simulink model "my_model"  (R2024a)
settings: Solver=VariableStepAuto  StartTime=0.0  StopTime=10.0  RelTol=1e-3
undefined symbols (not defined in the file): Kd, Kp, st0
settings Model: Creator=Qi Zhang  LastModifiedBy=dixiao
settings ConfigComp: CovBoundaryAbsTol=1.0e-5

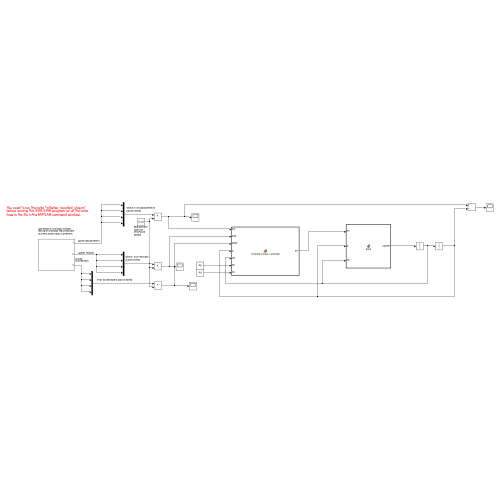
[thumbnail: Simulink's stored preview of the top-level diagram]
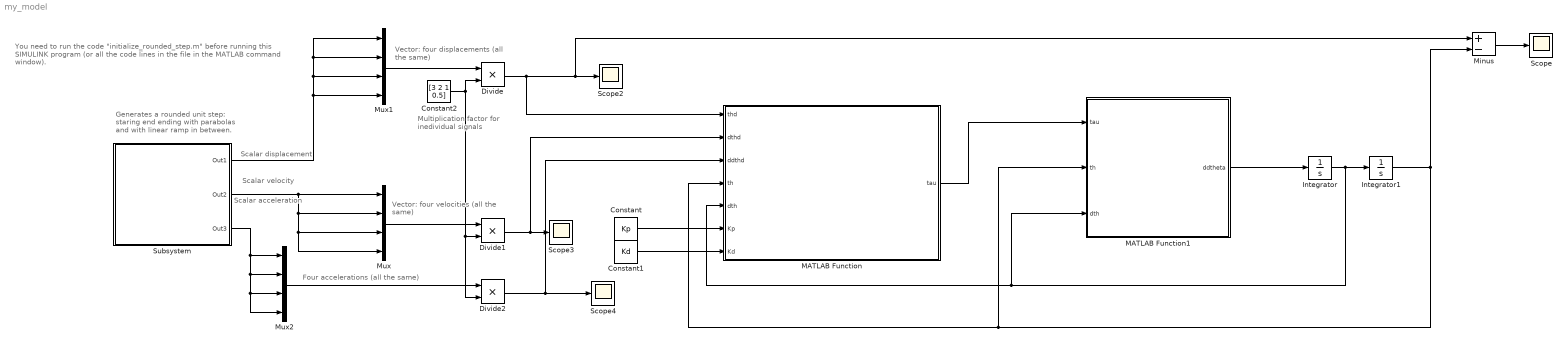
== system my_model ==
  note: You need to run the code "initialize_rounded_step.m"
      | before running this SIMULINK program (or all the code
      | lines in the file in the MATLAB command window).
  note: Generates a rounded unit step:
      | staring end ending with parabolas
      | and with linear ramp in between.
  note: Scalar velocity
  note: Four accelerations (all the same)
  note: Vector: four displacements
      | (all the same)
  note: Vector: four velocities
      | (all the same)
  note: Scalar displacement
  note: Multiplication
      | factor for
      | inedividual
      | signals
  note: Scalar
      | acceleration
  Constant : Constant  Value=Kp
  Constant1 : Constant  Value=Kd
  Constant2 : Constant  Value=[3 2 1 0.5]
  Divide : Product  Inputs=**
  Divide1 : Product  Inputs=**
  Divide2 : Product  Inputs=**
  Integrator : Integrator  InitialCondition=[0;0;0;0]
  Integrator1 : Integrator  InitialCondition=[0;0;0;0]
  MATLAB Function : MATLAB Function  TreatAsAtomicUnit=on
  MATLAB Function1 : MATLAB Function  TreatAsAtomicUnit=on
  Minus : Sum  Inputs=+-
  Mux : Mux
  Mux1 : Mux
  Mux2 : Mux
  Scope{,2..4} (4 alike) : Scope
  Subsystem : Subsystem
  wires:
  Subsystem/3(Out3) -> Mux2/2, Mux2/3, Mux2/4, Mux2/1
  Constant2/1 -> Divide2/2, Divide1/2, Divide/2
  Subsystem/2(Out2) -> Mux/4, Mux/3, Mux/2, Mux/1
  Mux1/1 -> Divide/1
  Divide/1 -> MATLAB Function/1(thd), Minus/1, Scope2/1
  Divide2/1 -> MATLAB Function/3(ddthd), Scope4/1
  Mux2/1 -> Divide2/1
  Mux/1 -> Divide1/1
  Subsystem/1(Out1) -> Mux1/1, Mux1/2, Mux1/3, Mux1/4
  Divide1/1 -> MATLAB Function/2(dthd), Scope3/1
  MATLAB Function1/1(ddtheta) -> Integrator/1
  Integrator/1 -> MATLAB Function1/3(dth), MATLAB Function/5(dth), Integrator1/1
  Constant/1 -> MATLAB Function/6(Kp)
  Constant1/1 -> MATLAB Function/7(Kd)
  Integrator1/1 -> Minus/2, MATLAB Function1/2(th), MATLAB Function/4(th)
  MATLAB Function/1(tau) -> MATLAB Function1/1(tau)
  Minus/1 -> Scope/1

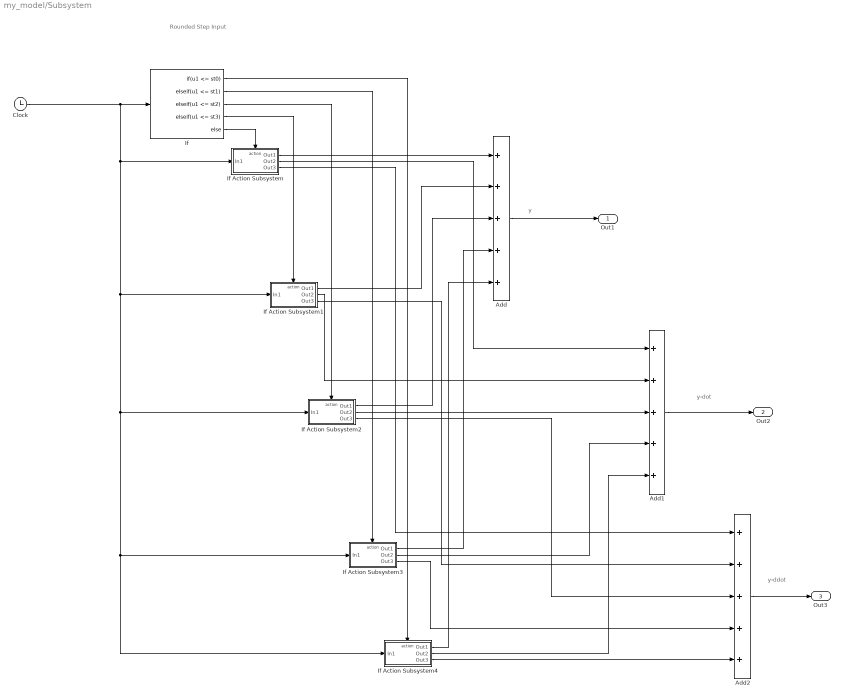
== system my_model/Subsystem ==
  note: Rounded Step Input
  note: y-ddot
  note: y-dot
  note: y
  Add : Sum  Inputs=+++++
  Add1 : Sum  Inputs=+++++
  Add2 : Sum  Inputs=+++++
  Clock : Clock
  If : If  IfExpression=u1 <= st0  ElseIfExpressions=u1 <= st1, u1 <= st2, u1 <= st3
  If Action Subsystem : Subsystem  TreatAsAtomicUnit=on
  If Action Subsystem1 : Subsystem  TreatAsAtomicUnit=on
  If Action Subsystem2 : Subsystem  TreatAsAtomicUnit=on
  If Action Subsystem3 : Subsystem  TreatAsAtomicUnit=on
  If Action Subsystem4 : Subsystem  TreatAsAtomicUnit=on
  Out1 : Outport
  Out2 : Outport  Port=2
  Out3 : Outport  Port=3
  wires:
  If Action Subsystem1/1(Out1) -> Add/2
  If/5 -> If Action Subsystem/Action
  If/3 -> If Action Subsystem2/Action
  If/2 -> If Action Subsystem3/Action
  If Action Subsystem/1(Out1) -> Add/1
  If Action Subsystem4/1(Out1) -> Add/5
  If/4 -> If Action Subsystem1/Action
  If/1 -> If Action Subsystem4/Action
  If Action Subsystem3/1(Out1) -> Add/4
  If Action Subsystem2/1(Out1) -> Add/3
  Add/1 -> Out1/1
  Add1/1 -> Out2/1
  Add2/1 -> Out3/1
  Clock/1 -> If Action Subsystem4/1(In1), If Action Subsystem3/1(In1), If Action Subsystem2/1(In1), If Action Subsystem1/1(In1), If Action Subsystem/1(In1), If/1
  If Action Subsystem/2(Out2) -> Add1/1
  If Action Subsystem/3(Out3) -> Add2/1
  If Action Subsystem1/2(Out2) -> Add1/2
  If Action Subsystem1/3(Out3) -> Add2/2
  If Action Subsystem2/2(Out2) -> Add1/3
  If Action Subsystem2/3(Out3) -> Add2/3
  If Action Subsystem3/3(Out3) -> Add2/4
  If Action Subsystem3/2(Out2) -> Add1/4
  If Action Subsystem4/2(Out2) -> Add1/5
  If Action Subsystem4/3(Out3) -> Add2/5

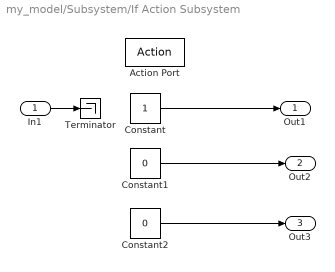
== system my_model/Subsystem/If Action Subsystem ==
  In1 : Inport
  Action Port : ActionPort  ActionPortLabel=else
  Constant : Constant
  Constant1 : Constant  Value=0
  Constant2 : Constant  Value=0
  Terminator : Terminator
  Out1 : Outport  OutputWhenDisabled=reset  InitialOutput=0
  Out2 : Outport  Port=2  OutputWhenDisabled=reset  InitialOutput=0
  Out3 : Outport  Port=3
  wires:
  Constant/1 -> Out1/1
  In1/1 -> Terminator/1
  Constant1/1 -> Out2/1
  Constant2/1 -> Out3/1

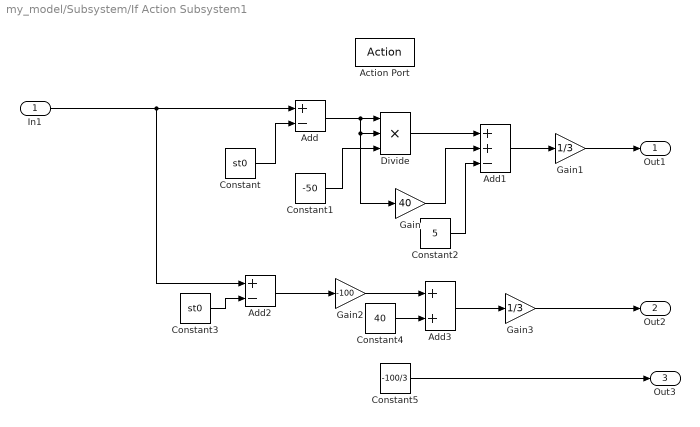
== system my_model/Subsystem/If Action Subsystem1 ==
  In1 : Inport
  Action Port : ActionPort  ActionPortLabel=elseif( u1 <= st3)
  Add : Sum  Inputs=+-
  Add1 : Sum  Inputs=++-
  Add2 : Sum  Inputs=+-
  Add3 : Sum
  Constant : Constant  Value=st0
  Constant1 : Constant  Value=-50
  Constant2 : Constant  Value=5
  Constant3 : Constant  Value=st0
  Constant4 : Constant  Value=40
  Constant5 : Constant  Value=-100/3
  Divide : Product  Inputs=***
  Gain : Gain  Gain=40
  Gain1 : Gain  Gain=1/3
  Gain2 : Gain  Gain=-100
  Gain3 : Gain  Gain=1/3
  Out1 : Outport  OutputWhenDisabled=reset  InitialOutput=0
  Out2 : Outport  Port=2  OutputWhenDisabled=reset  InitialOutput=0
  Out3 : Outport  Port=3  OutputWhenDisabled=reset  InitialOutput=0
  wires:
  In1/1 -> Add2/1, Add/1
  Constant1/1 -> Divide/3
  Constant/1 -> Add/2
  Add/1 -> Gain/1, Divide/2, Divide/1
  Divide/1 -> Add1/1
  Gain/1 -> Add1/2
  Constant2/1 -> Add1/3
  Add1/1 -> Gain1/1
  Gain1/1 -> Out1/1
  Add2/1 -> Gain2/1
  Gain2/1 -> Add3/1
  Add3/1 -> Gain3/1
  Constant3/1 -> Add2/2
  Constant4/1 -> Add3/2
  Gain3/1 -> Out2/1
  Constant5/1 -> Out3/1

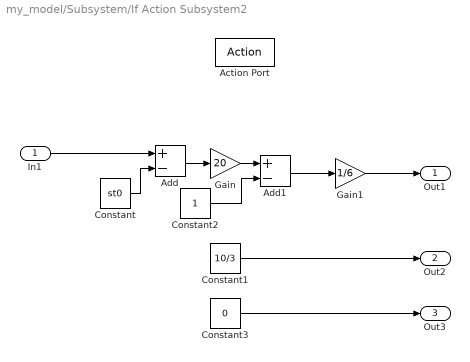
== system my_model/Subsystem/If Action Subsystem2 ==
  In1 : Inport
  Action Port : ActionPort  ActionPortLabel=elseif( u1 <= st2)
  Add : Sum  Inputs=+-
  Add1 : Sum  Inputs=+-
  Constant : Constant  Value=st0
  Constant1 : Constant  Value=10/3
  Constant2 : Constant
  Constant3 : Constant  Value=0
  Gain : Gain  Gain=20
  Gain1 : Gain  Gain=1/6
  Out1 : Outport  OutputWhenDisabled=reset  InitialOutput=0
  Out2 : Outport  Port=2  OutputWhenDisabled=reset  InitialOutput=0
  Out3 : Outport  Port=3  OutputWhenDisabled=reset  InitialOutput=0
  wires:
  In1/1 -> Add/1
  Constant/1 -> Add/2
  Add/1 -> Gain/1
  Gain/1 -> Add1/1
  Constant2/1 -> Add1/2
  Add1/1 -> Gain1/1
  Gain1/1 -> Out1/1
  Constant1/1 -> Out2/1
  Constant3/1 -> Out3/1

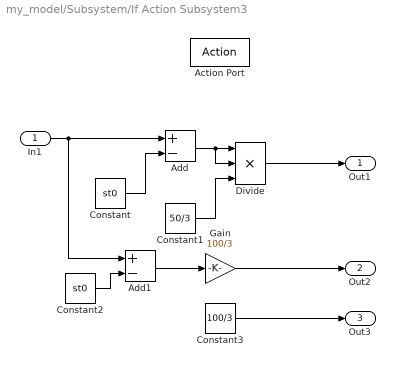
== system my_model/Subsystem/If Action Subsystem3 ==
  In1 : Inport
  Action Port : ActionPort  ActionPortLabel=elseif(u1 <= st1)
  Add : Sum  Inputs=+-
  Add1 : Sum  Inputs=+-
  Constant : Constant  Value=st0
  Constant1 : Constant  Value=50/3
  Constant2 : Constant  Value=st0
  Constant3 : Constant  Value=100/3
  Divide : Product  Inputs=***
  Gain : Gain  Gain=100/3
  Out1 : Outport  OutputWhenDisabled=reset  InitialOutput=0
  Out2 : Outport  Port=2  OutputWhenDisabled=reset  InitialOutput=0
  Out3 : Outport  Port=3  OutputWhenDisabled=reset  InitialOutput=0
  wires:
  In1/1 -> Add1/1, Add/1
  Constant/1 -> Add/2
  Add/1 -> Divide/2, Divide/1
  Constant1/1 -> Divide/3
  Divide/1 -> Out1/1
  Add1/1 -> Gain/1
  Constant2/1 -> Add1/2
  Gain/1 -> Out2/1
  Constant3/1 -> Out3/1

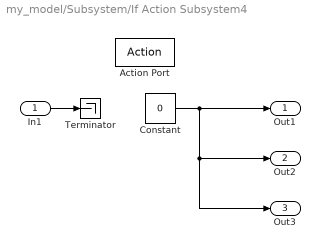
== system my_model/Subsystem/If Action Subsystem4 ==
  In1 : Inport
  Action Port : ActionPort  ActionPortLabel=if(u1 <= st0)
  Constant : Constant  Value=0
  Terminator : Terminator
  Out1 : Outport  OutputWhenDisabled=reset  InitialOutput=0
  Out2 : Outport  Port=2  OutputWhenDisabled=reset  InitialOutput=0
  Out3 : Outport  Port=3  OutputWhenDisabled=reset  InitialOutput=0
  wires:
  Constant/1 -> Out2/1, Out3/1, Out1/1
  In1/1 -> Terminator/1

== matlab function my_model/MATLAB Function1 ==
  data: tau input; ddtheta output; th input; dth input
function ddtheta = plant(tau,th,dth)
M = calc_M_fail(th);
C = calc_C_fail(th,dth);
N = calc_N_fail(th,dth);
ddtheta = inv(M)*(tau - C*dth-N);
end

== matlab function my_model/MATLAB Function ==
  data: thd input; tau output; dthd input; ddthd input; th input; dth input; Kp input; Kd input
function tau = compute_torque_controller(thd,dthd,ddthd,th,dth,Kp,Kd)
M = calc_M_fail(th);
C = calc_C_fail(th,dth);
N = calc_N_fail(th,dth);
e = thd - th;de = dthd - dth;
v = -Kd*de-Kp*e;
torque = M*ddthd+C*dth+N+M*v;

tau = torque;
end
